simulink model "Exp4Cdigital"  (R2015b)
settings: Solver=VariableStepAuto  StartTime=0.0  StopTime=0.7  RelTol=1e-5
undefined symbols (not defined in the file): DiscIntNeverNeededParam
libraries: dsparch4 x3, simulink x2
settings Model: Creator=mihai.ciobanu  LastModifiedBy=mihai.ciobanu
settings SolverCC: MaxConsecutiveMinStep=100

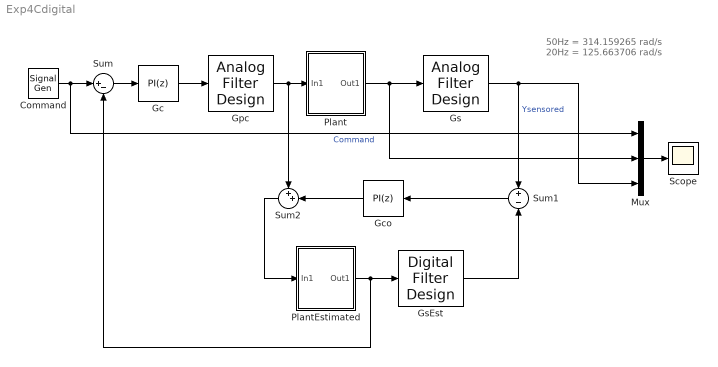
== system Exp4Cdigital ==
  note: 50Hz = 314.159265 rad/s
      | 20Hz = 125.663706 rad/s
  Command : SignalGenerator  WaveForm=square  Frequency=2
  Gc : simulink/Continuous/PID Controller  Controller=PI  TimeDomain=Discrete-time  SampleTime=0.001  IntegratorMethod=Trapezoidal  FilterMethod=Forward Euler  Form=Parallel  UseFilter=on  ControllerParametersSource=internal  P=1.5  I=30  D=0  N=100  InitialConditionSource=internal  InitialConditionForIntegrator=0  InitialConditionForFilter=0  ExternalReset=none  LimitOutput=off  UpperSaturationLimit=inf  LowerSaturationLimit=-inf  LinearizeAsGain=on  AntiWindupMode=none  Kb=1  TrackingMode=off  Kt=1  PParamMin=[]  PParamMax=[]  IParamMin=[]  IParamMax=[]  DParamMin=[]  DParamMax=[]  NParamMin=[]  NParamMax=[]  KbParamMin=[]  KbParamMax=[]  KtParamMin=[]  KtParamMax=[]  POutMin=[]  POutMax=[]  IOutMin=[]  IOutMax=[]  DOutMin=[]  DOutMax=[]  NOutMin=[]  NOutMax=[]  KbOutMin=[]  KbOutMax=[]  KtOutMin=[]  KtOutMax=[]  IntegratorOutMin=[]  IntegratorOutMax=[]  FilterOutMin=[]  FilterOutMax=[]  SumOutMin=[]  SumOutMax=[]  SumI1OutMin=[]  SumI1OutMax=[]  SumI2OutMin=[]  SumI2OutMax=[]  SumI3OutMin=[]  SumI3OutMax=[]  SumDOutMin=[]  SumDOutMax=[]  SaturationOutMin=[]  SaturationOutMax=[]  IntegratorContinuousStateAttributes=''  IntegratorStateMustResolveToSignalObject=off  IntegratorRTWStateStorageClass=Auto  FilterContinuousStateAttributes=''  FilterStateMustResolveToSignalObject=off  FilterRTWStateStorageClass=Auto  DifferentiatorICPrevScaledInput=0  DifferentiatorOutMin=[]  DifferentiatorOutMax=[]
  Gco : simulink/Continuous/PID Controller  Controller=PI  TimeDomain=Discrete-time  SampleTime=0.001  IntegratorMethod=Trapezoidal  FilterMethod=Forward Euler  Form=Parallel  UseFilter=on  ControllerParametersSource=internal  P=1.5  I=30  D=0  N=100  InitialConditionSource=internal  InitialConditionForIntegrator=0  InitialConditionForFilter=0  ExternalReset=none  LimitOutput=off  UpperSaturationLimit=inf  LowerSaturationLimit=-inf  LinearizeAsGain=on  AntiWindupMode=none  Kb=1  TrackingMode=off  Kt=1  PParamMin=[]  PParamMax=[]  IParamMin=[]  IParamMax=[]  DParamMin=[]  DParamMax=[]  NParamMin=[]  NParamMax=[]  KbParamMin=[]  KbParamMax=[]  KtParamMin=[]  KtParamMax=[]  POutMin=[]  POutMax=[]  IOutMin=[]  IOutMax=[]  DOutMin=[]  DOutMax=[]  NOutMin=[]  NOutMax=[]  KbOutMin=[]  KbOutMax=[]  KtOutMin=[]  KtOutMax=[]  IntegratorOutMin=[]  IntegratorOutMax=[]  FilterOutMin=[]  FilterOutMax=[]  SumOutMin=[]  SumOutMax=[]  SumI1OutMin=[]  SumI1OutMax=[]  SumI2OutMin=[]  SumI2OutMax=[]  SumI3OutMin=[]  SumI3OutMax=[]  SumDOutMin=[]  SumDOutMax=[]  SaturationOutMin=[]  SaturationOutMax=[]  IntegratorContinuousStateAttributes=''  IntegratorStateMustResolveToSignalObject=off  IntegratorRTWStateStorageClass=Auto  FilterContinuousStateAttributes=''  FilterStateMustResolveToSignalObject=off  FilterRTWStateStorageClass=Auto  DifferentiatorICPrevScaledInput=0  DifferentiatorOutMin=[]  DifferentiatorOutMax=[]
  Gpc : dsparch4/Analog Filter Design  method=Butterworth  filttype=Lowpass  N=2  Wlo=314.159265  Whi=80  Rp=2  Rs=40
  Gs : dsparch4/Analog Filter Design  method=Butterworth  filttype=Lowpass  N=1  Wlo=125.663706  Whi=80  Rp=2  Rs=40
  GsEst : dsparch4/Digital Filter Design  mwdsp_browser_bugfix_var=off
  Mux : Mux  Inputs=3
  Plant : Subsystem
  PlantEstimated : Subsystem
  Scope : Scope
  Sum : Sum  Inputs=|+-
  Sum1 : Sum  Inputs=+|-
  Sum2 : Sum  Inputs=++|
  wires:
  Sum/1 -> Gc/1
  Gc/1 -> Gpc/1
  Mux/1 -> Scope/1
  Command/1 -> Mux/1, Sum/1  "Command"
  Plant/1(Out1) -> Mux/2, Gs/1
  Gpc/1 -> Sum2/1, Plant/1(In1)
  Gs/1 -> Mux/3, Sum1/1  "Ysensored"
  Sum1/1 -> Gco/1
  Gco/1 -> Sum2/2
  Sum2/1 -> PlantEstimated/1(In1)
  GsEst/1 -> Sum1/2
  PlantEstimated/1(Out1) -> GsEst/1, Sum/2

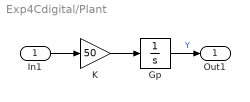
== system Exp4Cdigital/Plant ==
  In1 : Inport
  Gp : Integrator
  K : Gain  Gain=50
  Out1 : Outport
  wires:
  K/1 -> Gp/1
  In1/1 -> K/1
  Gp/1 -> Out1/1  "Y"

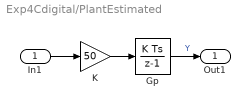
== system Exp4Cdigital/PlantEstimated ==
  In1 : Inport
  Gp : DiscreteIntegrator  InitialConditionSetting=State (most efficient)  SampleTime=0.001  ICPrevOutput=DiscIntNeverNeededParam  ICPrevScaledInput=DiscIntNeverNeededParam
  K : Gain  Gain=50
  Out1 : Outport
  wires:
  K/1 -> Gp/1
  In1/1 -> K/1
  Gp/1 -> Out1/1  "Y"
